simulink model "PRTS"  (R2021a)
settings: Solver=VariableStepAuto  StartTime=0.0  StopTime=200  RelTol=1e-3
settings Model: Creator=CFRPG  LastModifiedBy=CFRPG

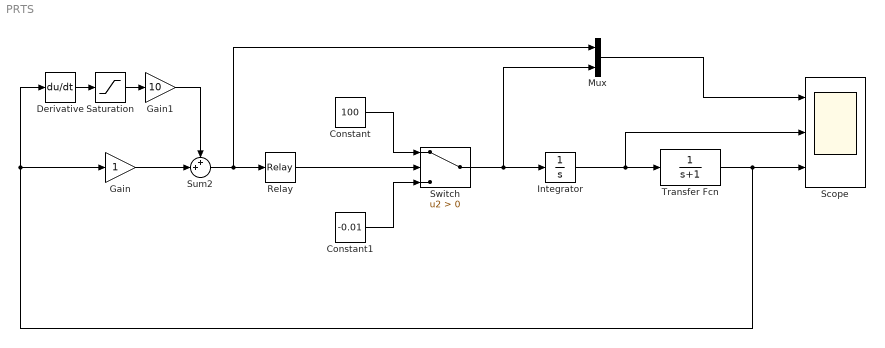
== system PRTS ==
  Constant : Constant  Value=100
  Constant1 : Constant  Value=-0.01
  Derivative : Derivative
  Gain : Gain
  Gain1 : Gain  Gain=10
  Integrator : Integrator
  Mux : Mux  Inputs=2
  Relay : Relay  OnSwitchValue=1  OffSwitchValue=0.3  OnOutputValue=0  OffOutputValue=1
  Saturation : Saturate  UpperLimit=10  LowerLimit=0
  Scope : Scope  NumInputPorts=3
  Sum2 : Sum  Inputs=++|
  Switch : Switch  Criteria=u2 > Threshold
  Transfer Fcn : TransferFcn  Denominator=[1 1]
  wires:
  Integrator/1 -> Scope/2, Transfer Fcn/1
  Transfer Fcn/1 -> Derivative/1, Gain/1, Scope/3
  Switch/1 -> Mux/2, Integrator/1
  Constant1/1 -> Switch/3
  Constant/1 -> Switch/1
  Relay/1 -> Switch/2
  Mux/1 -> Scope/1
  Derivative/1 -> Saturation/1
  Gain1/1 -> Sum2/1
  Saturation/1 -> Gain1/1
  Gain/1 -> Sum2/2
  Sum2/1 -> Relay/1, Mux/1
